simulink model "UPS_sim"  (R2016a)
settings: Solver=FixedStepAuto  StartTime=0.0  StopTime=sim_time  FixedStep=t_step  RelTol=1e-3
values from neighbouring files (symbols this model uses):
  dCez2 = Cez2.den{1}    [UPS_1data_experiment.m]    (also in UPS_3closedLoop.m)
  dCez3 = Cez3.den{1}    [UPS_1data_experiment.m]    (also in UPS_3closedLoop.m)
  dCiz2 = Ciz2.den{1}    [UPS_1data_experiment.m]    (also in UPS_3closedLoop.m)
  dCiz3 = Ciz3.den{1}    [UPS_1data_experiment.m]    (also in UPS_3closedLoop.m)
  dCz1 = Cz1.den{1}    [UPS_1data_experiment.m]    (also in UPS_2design5.m; UPS_3closedLoop.m)
  enRect = 0    [UPS_1data_experiment.m]    (also in UPS_3closedLoop.m)
  LoadType = 0    [UPS_1data_experiment.m]    (also in UPS_3closedLoop.m)
  ma = (Vopk)/Vin    [UPS_1data_experiment.m]    (also in UPS_3closedLoop.m = Vopk/Vin)
  nCez2 = Cez2.num{1}    [UPS_1data_experiment.m]    (also in UPS_3closedLoop.m)
  nCez3 = Cez3.num{1}    [UPS_1data_experiment.m]    (also in UPS_3closedLoop.m)
  nCiz2 = Ciz2.num{1}    [UPS_1data_experiment.m]    (also in UPS_3closedLoop.m)
  nCiz3 = Ciz3.num{1}    [UPS_1data_experiment.m]    (also in UPS_3closedLoop.m)
  nCz1 = Cz1.num{1}    [UPS_1data_experiment.m]    (also in UPS_2design5.m; UPS_3closedLoop.m)
  sel_control = 0    [UPS_1data_experiment.m]    (also in UPS_3closedLoop.m = 1)
  t_step = Ts/1000    (= 5e-08)    [UPS_1data_experiment.m]    (also in UPS_3closedLoop.m = 5e-07)
  Ta = 1/fa    (= 5e-05)    [UPS_1data_experiment.m]    (also in UPS_3closedLoop.m; test_hinf_norm.m; vrft_cascade_standard.m = Tde.Ts; vrft_flexible.m = Td.Ts)
  tload_down = 1    [UPS_1data_experiment.m]    (also in UPS_3closedLoop.m = 0.035)
  tload_up = 1    [UPS_1data_experiment.m]    (also in UPS_3closedLoop.m = 0.025)
  Vopk = 127*sqrt(2)    [UPS_1data_experiment.m]    (also in UPS_3closedLoop.m)
settings Model: Creator=Chrystian  LastModifiedBy=EKupa

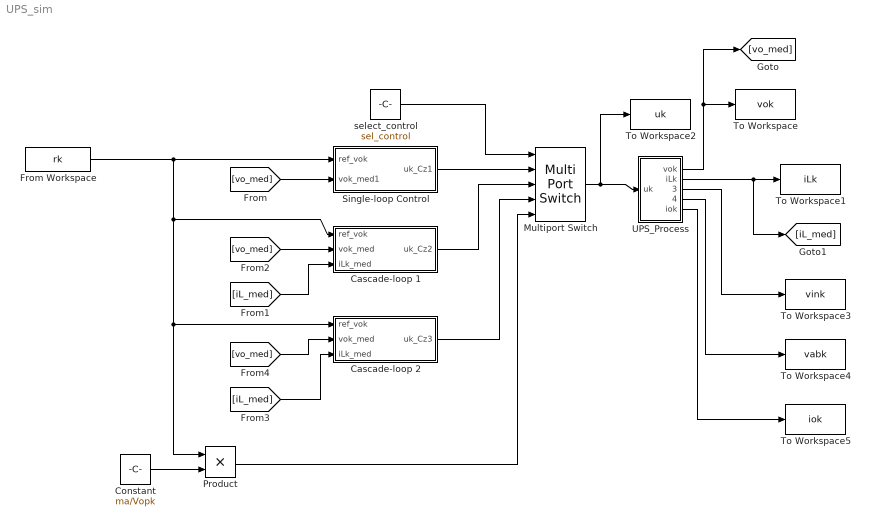
== system UPS_sim ==
  Cascade-loop 1 : Subsystem
  Cascade-loop 2 : Subsystem
  Constant : Constant  Value=ma/Vopk  SampleTime=Ta
  From Workspace : FromWorkspace  VariableName=rk  SampleTime=Ta
  Multiport Switch : MultiPortSwitch  DataPortForDefault=Additional data port  DiagnosticForDefault=None
  Product : Product
  Single-loop Control : Subsystem
  To Workspace : ToWorkspace  VariableName=vok  SampleTime=Ta
      settings: Save2DSignal=2-D array (concatenate along first dimension)
  To Workspace1 : ToWorkspace  VariableName=iLk  SampleTime=Ta
      settings: Save2DSignal=2-D array (concatenate along first dimension)
  To Workspace2 : ToWorkspace  VariableName=uk  SampleTime=Ta
      settings: Save2DSignal=2-D array (concatenate along first dimension)
  To Workspace3 : ToWorkspace  VariableName=vink  SampleTime=Ta
      settings: Save2DSignal=2-D array (concatenate along first dimension)
  To Workspace4 : ToWorkspace  VariableName=vabk  SampleTime=Ta
      settings: Save2DSignal=2-D array (concatenate along first dimension)
  To Workspace5 : ToWorkspace  VariableName=iok  SampleTime=Ta
      settings: Save2DSignal=2-D array (concatenate along first dimension)
  UPS_Process : Subsystem
  select_control : Constant  Value=sel_control  SampleTime=Ta
  wires:
  Single-loop Control/1(uk_Cz1) -> Multiport Switch/2
  Cascade-loop 1/1(uk_Cz2) -> Multiport Switch/3
  Cascade-loop 2/1(uk_Cz3) -> Multiport Switch/4
  select_control/1 -> Multiport Switch/1
  Multiport Switch/1 -> To Workspace2/1, UPS_Process/1(uk)
  UPS_Process/1(vok) -> [vo_med], To Workspace/1
  UPS_Process/2(iLk) -> [iL_med], To Workspace1/1
  [vo_med] -> Single-loop Control/2(vok_med1)
  [iL_med] -> Cascade-loop 1/3(iLk_med)
  [vo_med] -> Cascade-loop 1/2(vok_med)
  [vo_med] -> Cascade-loop 2/2(vok_med)
  [iL_med] -> Cascade-loop 2/3(iLk_med)
  UPS_Process/3(vink) -> To Workspace3/1
  UPS_Process/4(vabk) -> To Workspace4/1
  UPS_Process/5(iok) -> To Workspace5/1
  From Workspace/1 -> Single-loop Control/1(ref_vok), Product/1, Cascade-loop 2/1(ref_vok), Cascade-loop 1/1(ref_vok)
  Constant/1 -> Product/2
  Product/1 -> Multiport Switch/5

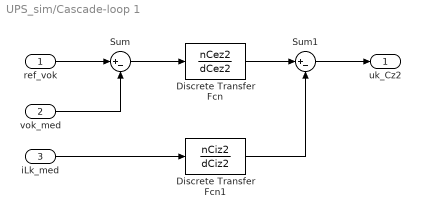
== system UPS_sim/Cascade-loop 1 ==
  ref_vok : Inport
  vok_med : Inport  Port=2
  iLk_med : Inport  Port=3
  Discrete Transfer Fcn : DiscreteTransferFcn  Numerator=nCez2  Denominator=dCez2  SampleTime=Ta
  Discrete Transfer Fcn1 : DiscreteTransferFcn  Numerator=nCiz2  Denominator=dCiz2  SampleTime=Ta
  Sum : Sum  Inputs=|+-
  Sum1 : Sum  Inputs=|+-
  uk_Cz2 : Outport
  wires:
  Sum/1 -> Discrete Transfer Fcn/1
  vok_med/1 -> Sum/2
  ref_vok/1 -> Sum/1
  iLk_med/1 -> Discrete Transfer Fcn1/1
  Discrete Transfer Fcn/1 -> Sum1/1
  Sum1/1 -> uk_Cz2/1
  Discrete Transfer Fcn1/1 -> Sum1/2

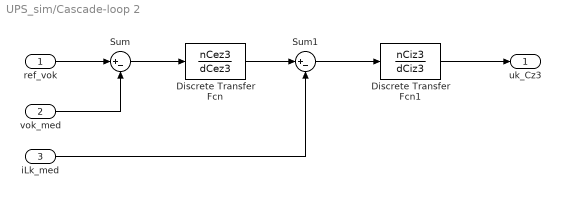
== system UPS_sim/Cascade-loop 2 ==
  ref_vok : Inport
  vok_med : Inport  Port=2
  iLk_med : Inport  Port=3
  Discrete Transfer Fcn : DiscreteTransferFcn  Numerator=nCez3  Denominator=dCez3  SampleTime=Ta
  Discrete Transfer Fcn1 : DiscreteTransferFcn  Numerator=nCiz3  Denominator=dCiz3  SampleTime=Ta
  Sum : Sum  Inputs=|+-
  Sum1 : Sum  Inputs=|+-
  uk_Cz3 : Outport
  wires:
  Sum/1 -> Discrete Transfer Fcn/1
  vok_med/1 -> Sum/2
  ref_vok/1 -> Sum/1
  Discrete Transfer Fcn/1 -> Sum1/1
  Sum1/1 -> Discrete Transfer Fcn1/1
  Discrete Transfer Fcn1/1 -> uk_Cz3/1
  iLk_med/1 -> Sum1/2

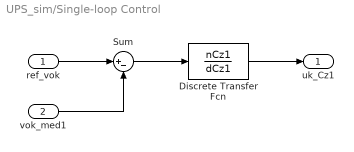
== system UPS_sim/Single-loop Control ==
  ref_vok : Inport
  vok_med1 : Inport  Port=2
  Discrete Transfer Fcn : DiscreteTransferFcn  Numerator=nCz1  Denominator=dCz1  SampleTime=Ta
  Sum : Sum  Inputs=|+-
  uk_Cz1 : Outport
  wires:
  Sum/1 -> Discrete Transfer Fcn/1
  Discrete Transfer Fcn/1 -> uk_Cz1/1
  vok_med1/1 -> Sum/2
  ref_vok/1 -> Sum/1

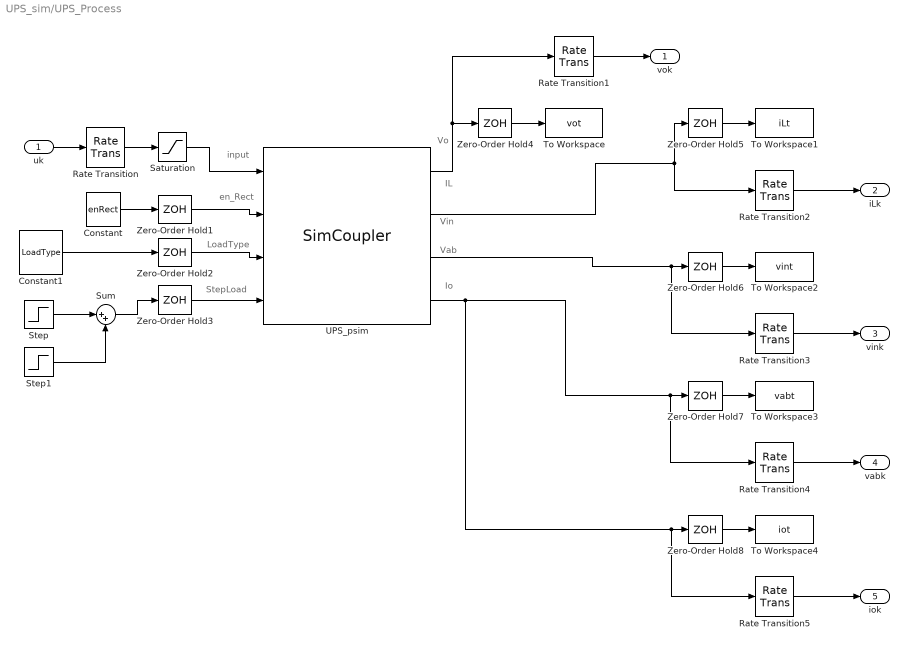
== system UPS_sim/UPS_Process ==
  note: IL
  note: Vo
  note: StepLoad
  note: LoadType
  note: en_Rect
  note: input
  note: Vin
  note: Vab
  note: Io
  uk : Inport
  Constant : Constant  Value=enRect  SampleTime=t_step
  Constant1 : Constant  Value=LoadType  SampleTime=t_step
  Rate Transition : RateTransition  Deterministic=off  OutPortSampleTime=t_step
  Rate Transition{1..5} (5 alike) : RateTransition  OutPortSampleTime=Ta
  Saturation : Saturate  UpperLimit=1  LowerLimit=-1
  Step : Step  Time=tload_up  SampleTime=t_step
  Step1 : Step  Time=tload_down  After=-1  SampleTime=t_step
  Sum : Sum  Inputs=|++
  To Workspace : ToWorkspace  VariableName=vot  SampleTime=t_step
      settings: Save2DSignal=2-D array (concatenate along first dimension)
  To Workspace1 : ToWorkspace  VariableName=iLt  SampleTime=t_step
      settings: Save2DSignal=2-D array (concatenate along first dimension)
  To Workspace2 : ToWorkspace  VariableName=vint  SampleTime=t_step
      settings: Save2DSignal=2-D array (concatenate along first dimension)
  To Workspace3 : ToWorkspace  VariableName=vabt  SampleTime=t_step
      settings: Save2DSignal=2-D array (concatenate along first dimension)
  To Workspace4 : ToWorkspace  VariableName=iot  SampleTime=t_step
      settings: Save2DSignal=2-D array (concatenate along first dimension)
  UPS_psim : S-Function  FunctionName=SimCoupler  Parameters='C:\Users\EKupa\Downloads\UPS - R2\UPS_psim.psimsch'  SFunctionDeploymentMode=off  EnableBusSupport=off
      mask init:
      | c=[0:10:360]*pi/180;
      | x1=cos(c)*30; y1=sin(c)*30+20;
      | x2=cos(c)*30;y2=sin(c)*30-20;
      settings: OpenFcn=PSimDialog('PSimFileEdt','Value','Parameters');  CloseFcn=close(gcf);
      mask Display: plot(-60,-60,60,60,x1,y1,x2,y2)
  Zero-Order Hold{1..8} (8 alike) : ZeroOrderHold  SampleTime=t_step
  vok : Outport
  iLk : Outport  Port=2
  vink : Outport  Port=3
  vabk : Outport  Port=4
  iok : Outport  Port=5
  wires:
  Step/1 -> Sum/1
  Constant1/1 -> Zero-Order Hold2/1
  Zero-Order Hold1/1 -> UPS_psim/2
  Zero-Order Hold4/1 -> To Workspace/1
  Step1/1 -> Sum/2
  Zero-Order Hold2/1 -> UPS_psim/3
  UPS_psim/1 -> Rate Transition1/1, Zero-Order Hold4/1
  Zero-Order Hold3/1 -> UPS_psim/4
  Constant/1 -> Zero-Order Hold1/1
  Sum/1 -> Zero-Order Hold3/1
  UPS_psim/2 -> Zero-Order Hold5/1, Rate Transition2/1
  Zero-Order Hold5/1 -> To Workspace1/1
  Rate Transition1/1 -> vok/1
  Rate Transition2/1 -> iLk/1
  uk/1 -> Rate Transition/1
  Zero-Order Hold6/1 -> To Workspace2/1
  Rate Transition3/1 -> vink/1
  UPS_psim/3 -> Rate Transition3/1, Zero-Order Hold6/1
  Zero-Order Hold7/1 -> To Workspace3/1
  Rate Transition4/1 -> vabk/1
  Zero-Order Hold8/1 -> To Workspace4/1
  Rate Transition5/1 -> iok/1
  UPS_psim/4 -> Rate Transition5/1, Zero-Order Hold8/1, Rate Transition4/1, Zero-Order Hold7/1
  Rate Transition/1 -> Saturation/1
  Saturation/1 -> UPS_psim/1
